simulink model "examples_from_book"  (R2023b)
settings: Solver=ode4  StartTime=0.0  StopTime=0.16  MaxStep=1e-6  RelTol=1e-4  AbsTol=1e-6
libraries: spsParallelRLCBranchLib x20, spsIGBTDiodeLib x6, spsGroundLib x5, spsThreePhaseVIMeasurementLib x3, spsTriangleGeneratorLib x3, spsCurrentMeasurementLib x2, spsDCVoltageSourceLib x2, spsVoltageMeasurementLib x2, spsACVoltageSourceLib x1, spsControlledCurrentSourceLib x1, spsPowerLib x1, spsPower3phInstantaneousLib x1
settings Model: Creator=debatir  LastModifiedBy=debatir
settings SolverCC: SolverResetMethod=Robust

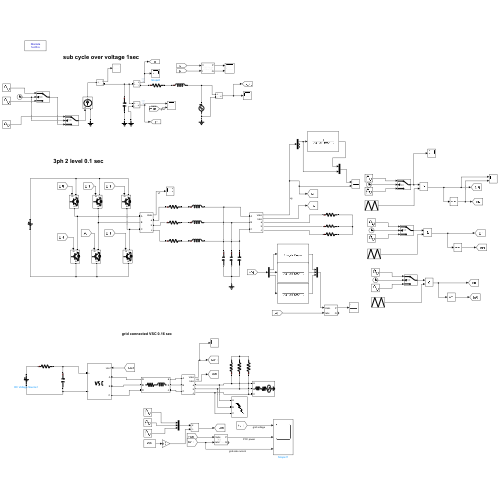
[thumbnail: Simulink's stored preview of the top-level diagram]
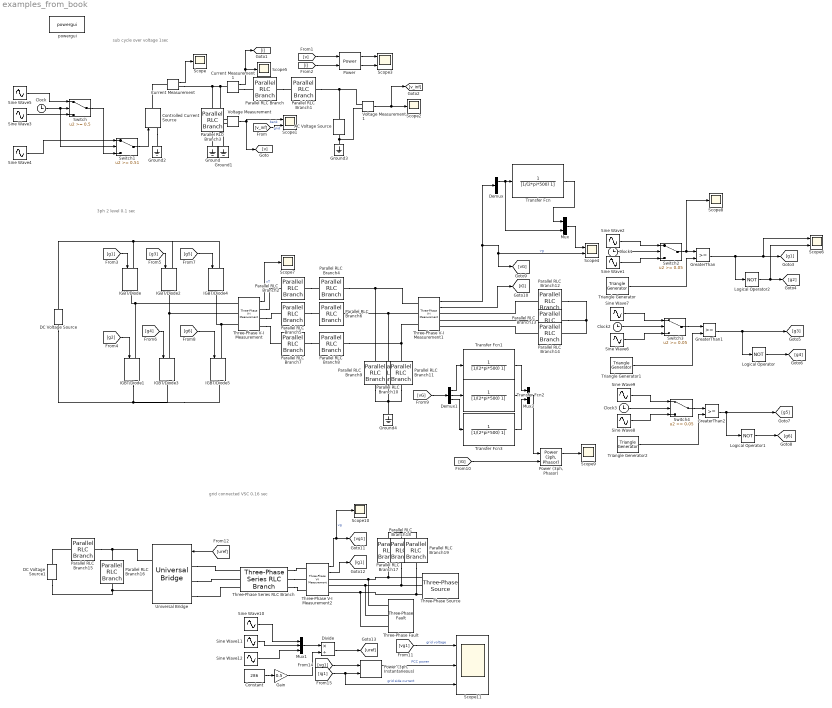
== system examples_from_book ==
  note: grid connected VSC 0.16 sec
  note: 3ph 2 level 0.1 sec
  note: sub cycle over voltage 1sec
  AC Voltage Source : spsACVoltageSourceLib/AC Voltage Source  Amplitude=1  Phase=0  Frequency=60  SampleTime=50e-6  Measurements=None  BusType=PV  Pref=10e3  Qref=0  Qmin=-inf  Qmax=+inf
  Clock{,1..3} (4 alike) : Clock
  Constant : Constant  Value=286
  Controlled Current Source : spsControlledCurrentSourceLib/Controlled Current Source  Initialize=on  Source_Type=AC  Amplitude=0  Phase=0  Frequency=0  Measurements=None
  Current Measurement : spsCurrentMeasurementLib/Current Measurement  PhasorSimulation=off  OutputType=Complex  PSBequivalent=0
  Current Measurement1 : spsCurrentMeasurementLib/Current Measurement  PhasorSimulation=off  OutputType=Complex  PSBequivalent=0
  DC Voltage Source : spsDCVoltageSourceLib/DC Voltage Source  Amplitude=282  Measurements=None
  DC Voltage Source1 : spsDCVoltageSourceLib/DC Voltage Source  Amplitude=286  Measurements=None
  Demux : Demux  Outputs=3
  Demux1 : Demux  Outputs=3
  Divide : Product  Inputs=*/
  Gain : Gain  Gain=0.5
  GreaterThan : RelationalOperator  OutDataTypeStr=boolean  RndMeth=Simplest  InputSameDT=off
  GreaterThan1 : RelationalOperator  OutDataTypeStr=boolean  RndMeth=Simplest  InputSameDT=off
  GreaterThan2 : RelationalOperator  OutDataTypeStr=boolean  RndMeth=Simplest  InputSameDT=off
  Ground{,1..4} (5 alike) : spsGroundLib/Ground  LConnTagsString=a
  IGBT/Diode{,1..5} (6 alike) : spsIGBTDiodeLib/IGBT//Diode  Ron=1e-3  Rs=1e5  Cs=inf  Measurements=off
  Logical Operator : Logic  Operator=NOT  AllPortsSameDT=off  OutDataTypeStr=boolean
  Logical Operator1 : Logic  Operator=NOT  AllPortsSameDT=off  OutDataTypeStr=boolean
  Logical Operator2 : Logic  Operator=NOT  AllPortsSameDT=off  OutDataTypeStr=boolean
  Mux : Mux  Inputs=2
  Mux1 : Mux  Inputs=3
  Mux3 : Mux  Inputs=3
  Parallel RLC Branch : spsParallelRLCBranchLib/Parallel RLC Branch  LConnTagsString=a  RConnTagsString=__new0  BranchType=R  Resistance=0.05  Inductance=0.05  SetiL0=off  InitialCurrent=0  Capacitance=1e-6  Setx0=off  InitialVoltage=0  Measurements=None
  Parallel RLC Branch1 : spsParallelRLCBranchLib/Parallel RLC Branch  LConnTagsString=a  RConnTagsString=__new0  BranchType=L  Resistance=1  Inductance=0.5/(2*pi*60)  SetiL0=off  InitialCurrent=0  Capacitance=1e-6  Setx0=off  InitialVoltage=0  Measurements=None
  Parallel RLC Branch10 : spsParallelRLCBranchLib/Parallel RLC Branch  LConnTagsString=a  RConnTagsString=__new0  BranchType=C  Resistance=1  Inductance=0.2/(2*pi*60)  SetiL0=off  InitialCurrent=0  Capacitance=30e-6  Setx0=off  InitialVoltage=0  Measurements=None
  Parallel RLC Branch11 : spsParallelRLCBranchLib/Parallel RLC Branch  LConnTagsString=a  RConnTagsString=__new0  BranchType=C  Resistance=1  Inductance=0.2/(2*pi*60)  SetiL0=off  InitialCurrent=0  Capacitance=30e-6  Setx0=off  InitialVoltage=0  Measurements=None
  Parallel RLC Branch{12..14,17..19} (6 alike) : spsParallelRLCBranchLib/Parallel RLC Branch  LConnTagsString=a  RConnTagsString=__new0  BranchType=R  Resistance=1  Inductance=0.05  SetiL0=off  InitialCurrent=0  Capacitance=1e-6  Setx0=off  InitialVoltage=0  Measurements=None
  Parallel RLC Branch15 : spsParallelRLCBranchLib/Parallel RLC Branch  LConnTagsString=a  RConnTagsString=__new0  BranchType=R  Resistance=0.05  Inductance=0.05  SetiL0=off  InitialCurrent=0  Capacitance=1e-6  Setx0=off  InitialVoltage=0  Measurements=None
  Parallel RLC Branch16 : spsParallelRLCBranchLib/Parallel RLC Branch  LConnTagsString=a  RConnTagsString=__new0  BranchType=C  Resistance=1  Inductance=0.2/(2*pi*60)  SetiL0=off  InitialCurrent=0  Capacitance=0.09  Setx0=off  InitialVoltage=0  Measurements=None
  Parallel RLC Branch2 : spsParallelRLCBranchLib/Parallel RLC Branch  LConnTagsString=a  RConnTagsString=__new0  BranchType=R  Resistance=0.02  Inductance=0.05  SetiL0=off  InitialCurrent=0  Capacitance=1e-6  Setx0=off  InitialVoltage=0  Measurements=None
  Parallel RLC Branch3 : spsParallelRLCBranchLib/Parallel RLC Branch  LConnTagsString=a  RConnTagsString=__new0  BranchType=C  Resistance=1  Inductance=0.2/(2*pi*60)  SetiL0=off  InitialCurrent=0  Capacitance=0.2/(2*pi*60)  Setx0=off  InitialVoltage=0  Measurements=None
  Parallel RLC Branch4 : spsParallelRLCBranchLib/Parallel RLC Branch  LConnTagsString=a  RConnTagsString=__new0  BranchType=L  Resistance=1  Inductance=0.003  SetiL0=off  InitialCurrent=0  Capacitance=1e-6  Setx0=off  InitialVoltage=0  Measurements=None
  Parallel RLC Branch5 : spsParallelRLCBranchLib/Parallel RLC Branch  LConnTagsString=a  RConnTagsString=__new0  BranchType=R  Resistance=0.02  Inductance=0.05  SetiL0=off  InitialCurrent=0  Capacitance=1e-6  Setx0=off  InitialVoltage=0  Measurements=None
  Parallel RLC Branch6 : spsParallelRLCBranchLib/Parallel RLC Branch  LConnTagsString=a  RConnTagsString=__new0  BranchType=L  Resistance=1  Inductance=0.003  SetiL0=off  InitialCurrent=0  Capacitance=1e-6  Setx0=off  InitialVoltage=0  Measurements=None
  Parallel RLC Branch7 : spsParallelRLCBranchLib/Parallel RLC Branch  LConnTagsString=a  RConnTagsString=__new0  BranchType=R  Resistance=0.02  Inductance=0.05  SetiL0=off  InitialCurrent=0  Capacitance=1e-6  Setx0=off  InitialVoltage=0  Measurements=None
  Parallel RLC Branch8 : spsParallelRLCBranchLib/Parallel RLC Branch  LConnTagsString=a  RConnTagsString=__new0  BranchType=L  Resistance=1  Inductance=0.003  SetiL0=off  InitialCurrent=0  Capacitance=1e-6  Setx0=off  InitialVoltage=0  Measurements=None
  Parallel RLC Branch9 : spsParallelRLCBranchLib/Parallel RLC Branch  LConnTagsString=a  RConnTagsString=__new0  BranchType=C  Resistance=1  Inductance=0.2/(2*pi*60)  SetiL0=off  InitialCurrent=0  Capacitance=30e-6  Setx0=off  InitialVoltage=0  Measurements=None
  Power : spsPowerLib/Power  Freq=60  Vinit=[1, 0]  Iinit=[1, 0]  Ts=0
  "Power (3ph, Instantaneous)" : spsPower3phInstantaneousLib/Power (3ph, Instantaneous)
  "Power (3ph, Phasor)" : spsPower3phPhasorLib/Power (3ph, Phasor)
      settings: LibrarySourceBlock=|
      | sps_lib/Sensors and Measurements/Power
      | (3ph, Phasor)
  Scope{,2,5,7..10} (7 alike) : Scope
  Scope{1,3..4,6} (4 alike) : Scope  NumInputPorts=2
  Scope11 : Scope  NumInputPorts=3
  Sine Wave1 : Sin  Frequency=376.991118  SampleTime=1e-6
  Sine Wave10 : Sin  Amplitude=163  Frequency=376.991118  SampleTime=1e-6
  Sine Wave11 : Sin  Amplitude=163  Frequency=376.991118  Phase=4.18879  SampleTime=1e-6
  Sine Wave12 : Sin  Amplitude=163  Frequency=376.991118  Phase=(2*pi)/3  SampleTime=1e-6
  Sine Wave2 : Sin  Amplitude=.8  Frequency=376.991118  SampleTime=1e-6
  Sine Wave3 : Sin  Frequency=376.991118  SampleTime=50e-6
  Sine Wave4 : Sin  Amplitude=0  Frequency=376.991118  SampleTime=50e-6
  Sine Wave5 : Sin  Amplitude=0.5  Frequency=376.991118  SampleTime=50e-6
  Sine Wave6 : Sin  Frequency=376.991118  Phase=4.18879  SampleTime=1e-6
  Sine Wave7 : Sin  Amplitude=.8  Frequency=376.991118  Phase=4.18879  SampleTime=1e-6
  Sine Wave8 : Sin  Frequency=376.991118  Phase=(2*pi)/3  SampleTime=1e-6
  Sine Wave9 : Sin  Amplitude=.8  Frequency=376.991118  Phase=(2*pi)/3  SampleTime=1e-6
  Switch : Switch  Threshold=0.5  SaturateOnIntegerOverflow=off  InputSameDT=off
  Switch1 : Switch  Threshold=0.51  SaturateOnIntegerOverflow=off  InputSameDT=off
  Switch2 : Switch  Threshold=0.05  SaturateOnIntegerOverflow=off  InputSameDT=off
  Switch3 : Switch  Threshold=0.05  SaturateOnIntegerOverflow=off  InputSameDT=off
  Switch4 : Switch  Threshold=0.05  SaturateOnIntegerOverflow=off  InputSameDT=off
  Three-Phase Series RLC Branch : spsThreePhaseSeriesRLCBranchLib/Three-Phase Series RLC Branch  LConnTagsString=A|B|C  RConnTagsString=A|B|C  BranchType=RL  Resistance=0.016  Inductance=0.2122e-3  Capacitance=1e-6  Measurements=None
  Three-Phase V-I Measurement : spsThreePhaseVIMeasurementLib/Three-Phase V-I Measurement  VoltageMeasurement=phase-to-ground  SetLabelV=off  LabelV=Vabc  Vpu=off  VpuLL=off  CurrentMeasurement=no  SetLabelI=off  LabelI=Iabc  Ipu=off  Pbase=100e6  Vbase=500e3  OutputType=Complex  PhasorSimulation=off  PSBequivalent=0
  Three-Phase V-I Measurement1 : spsThreePhaseVIMeasurementLib/Three-Phase V-I Measurement  VoltageMeasurement=phase-to-ground  SetLabelV=off  LabelV=Vabc  Vpu=off  VpuLL=off  CurrentMeasurement=yes  SetLabelI=off  LabelI=Iabc  Ipu=off  Pbase=100e6  Vbase=500e3  OutputType=Complex  PhasorSimulation=off  PSBequivalent=0
  Three-Phase V-I Measurement2 : spsThreePhaseVIMeasurementLib/Three-Phase V-I Measurement  VoltageMeasurement=phase-to-ground  SetLabelV=off  LabelV=Vabc  Vpu=off  VpuLL=off  CurrentMeasurement=yes  SetLabelI=off  LabelI=Iabc  Ipu=off  Pbase=10e6  Vbase=400  OutputType=Complex  PhasorSimulation=off  PSBequivalent=0
  Three-Phase Fault : spsThreePhaseFaultLib/Three-Phase Fault  InitialStates=0  FaultA=on  FaultB=on  FaultC=on  GroundFault=on  SwitchTimes="[0.05  0.05+3/60]"  External=off  SwitchStatus=NaN  FaultResistance=0.001  GroundResistance=0.01  SnubberResistance=1e6  SnubberCapacitance=inf  Measurements=None
  Three-Phase Source : spsThreePhaseSourceLib/Three-Phase Source  InternalConnection=Yg  VoltagePhases=off  Voltage=175  PhaseAngle=0  Voltage_phases=[25e3 25e3 25e3]/sqrt(3)  PhaseAngles_phases=[0 -120 +120]  Frequency=60  NonIdealSource=on  SpecifyImpedance=off  Resistance=1.6  Inductance=16.58e-3  ShortCircuitLevel=100e6  BaseVoltage=25e3  XRratio=7  BusType=swing  Pref=10e3  Qref=0  Prefabc=[10e3, 10e3, 10e3]  Qrefabc=[0, 0, 0]  Qmin=-inf  Qmax=inf
  Transfer Fcn{,1..3} (4 alike) : TransferFcn  Numerator=[0 1]  Denominator=[1/(2*pi*500) 1]
  Triangle Generator : spsTriangleGeneratorLib/Triangle Generator  Freq=1980  Phase=0  Ts=1e-6
  Triangle Generator1 : spsTriangleGeneratorLib/Triangle Generator  Freq=1980  Phase=0  Ts=1e-6
  Triangle Generator2 : spsTriangleGeneratorLib/Triangle Generator  Freq=1980  Phase=0  Ts=1e-6
  Universal Bridge : spsUniversalBridgeLib/Universal Bridge  Arms=3  SnubberResistance=1e5  SnubberCapacitance=inf  Device=Average-model based VSC  Ron=1e-3  Lon=0  ForwardVoltages="[  0  0  ]"  ForwardVoltage=0  GTOparameters=[ 10e-6 , 20e-6 ]  IGBTparameters=[ 1e-6 , 2e-6 ]  Measurements=None  Measurements_2=None  converterType=Rectifier
  Voltage Measurement : spsVoltageMeasurementLib/Voltage Measurement  PhasorSimulation=off  OutputType=Complex  PSBequivalent=0
  Voltage Measurement1 : spsVoltageMeasurementLib/Voltage Measurement  PhasorSimulation=off  OutputType=Complex  PSBequivalent=0
  powergui : sps_lib/powergui  Priority=1  SimulationMode=Discrete  SampleTime=1e-6  frequency=60  Iterations=50  frequencyindice=0  Pbase=100e6  ErrMax=1e-4  UnitsV=kV  UnitsW=MW  buscounter=0  FunctionMessages=off  echomessages=off  EnableUseOfTLC=off  CurrentSourceSwitches=off  DisableSnubberDevices=off  DisableRonSwitches=off  DisableVfSwitches=off  DisplayEquations=off  AutomaticDiscreteSolvers=off  SolverType=Tustin  Interpol=off  ExternalGateDelay=off  methode=off  Ts=100  x0status=blocks  SPID=on  SwTol=0  HookPort=off  NonlinearTolerance=1e-4  nMaxIteration=100  ContinueOnMaxIteration=off  RestoreLinks=warning  ResistiveCurrentMeasurement=off  Frange=[0:2:500]  Ylog=off  Xlog=on  ShowGrid=off  save=off  variable=ZData  structure=0  ZoomFFT=off  StartTime=0.0  cycles=1  DisplayStyle=1  fundamental=60  FreqAxis=off  MaxFrequency=1000  frequencyindicesteady=1  RmsSteady=1  display=off
  wires:
  Current Measurement/1 -> Scope/1
  Voltage Measurement/1 -> [v], Scope1/1  "bank"
  [v_inf] -> Scope1/2  "grid"
  Voltage Measurement1/1 -> [v_inf], Scope2/1
  [v] -> Power/1
  [i] -> Power/2
  Power/1 -> Scope3/1
  Power/2 -> Scope3/2
  Current Measurement1/1 -> [i], Scope5/1
  Clock/1 -> Switch1/2, Switch/2
  Sine Wave5/1 -> Switch/1
  Sine Wave3/1 -> Switch/3
  Switch1/1 -> Controlled Current Source/1
  Switch/1 -> Switch1/3
  Sine Wave4/1 -> Switch1/1
  Sine Wave1/1 -> Switch2/3
  Clock1/1 -> Switch2/2
  Sine Wave2/1 -> Switch2/1
  Triangle Generator/1 -> GreaterThan/2
  GreaterThan/1 -> Logical Operator2/1, Scope6/1, [g1]
  Logical Operator2/1 -> Scope6/2, [g2]
  Logical Operator/1 -> [g4]
  GreaterThan1/1 -> Logical Operator/1, [g3]
  Triangle Generator1/1 -> GreaterThan1/2
  Sine Wave7/1 -> Switch3/1
  Clock2/1 -> Switch3/2
  Sine Wave6/1 -> Switch3/3
  Sine Wave8/1 -> Switch4/3
  Clock3/1 -> Switch4/2
  Sine Wave9/1 -> Switch4/1
  Switch4/1 -> GreaterThan2/1
  Triangle Generator2/1 -> GreaterThan2/2
  GreaterThan2/1 -> [g5], Logical Operator1/1
  Logical Operator1/1 -> [g6]
  [g1] -> IGBT/Diode/1
  [g2] -> IGBT/Diode1/1
  [g3] -> IGBT/Diode2/1
  [g4] -> IGBT/Diode3/1
  [g5] -> IGBT/Diode4/1
  [g6] -> IGBT/Diode5/1
  Three-Phase V-I Measurement1/1 -> Demux/1, [vG], Scope4/2  "vg"
  Three-Phase V-I Measurement/1 -> Scope7/1  "vT"
  Switch3/1 -> GreaterThan1/1
  Switch2/1 -> Scope8/1, GreaterThan/1
  Three-Phase V-I Measurement1/2 -> [iG]
  [iG] -> "Power (3ph, Phasor)"/2
  "Power (3ph, Phasor)"/1 -> Scope9/1
  Demux/1 -> Mux/2, Transfer Fcn/1
  Transfer Fcn/1 -> Mux/1
  Mux/1 -> Scope4/1
  Three-Phase V-I Measurement2/2 -> [ig1]
  Three-Phase V-I Measurement2/1 -> Scope10/1, [vg1]  "vg"
  Constant/1 -> Gain/1
  Gain/1 -> Divide/2
  Divide/1 -> [uref]
  [uref] -> Universal Bridge/1
  Mux1/1 -> Divide/1
  Sine Wave10/1 -> Mux1/1
  Sine Wave11/1 -> Mux1/2
  Sine Wave12/1 -> Mux1/3
  [vg1] -> Scope11/1  "grid voltage"
  [vg1] -> "Power (3ph, Instantaneous)"/1
  [ig1] -> Scope11/3, "Power (3ph, Instantaneous)"/2  "grid side current"
  [vG] -> Demux1/1
  Demux1/1 -> Transfer Fcn1/1
  Demux1/2 -> Transfer Fcn2/1
  Demux1/3 -> Transfer Fcn3/1
  Transfer Fcn2/1 -> Mux3/2
  Transfer Fcn1/1 -> Mux3/1
  Transfer Fcn3/1 -> Mux3/3
  Mux3/1 -> "Power (3ph, Phasor)"/1
  "Power (3ph, Instantaneous)"/1 -> Scope11/2  "PCC power"
  connections:
  Parallel RLC Branch/RConn1 -- Parallel RLC Branch1/LConn1
  Current Measurement/RConn1 -- Parallel RLC Branch3/LConn1 -- Current Measurement1/LConn1 -- Voltage Measurement/LConn1
  Controlled Current Source/RConn1 -- Current Measurement/LConn1
  Ground/LConn1 -- Parallel RLC Branch3/RConn1
  Ground1/LConn1 -- Voltage Measurement/LConn2
  Controlled Current Source/LConn1 -- Ground2/LConn1
  Parallel RLC Branch1/RConn1 -- Voltage Measurement1/LConn1 -- AC Voltage Source/RConn1
  Ground3/LConn1 -- Voltage Measurement1/LConn2 -- AC Voltage Source/LConn1
  Current Measurement1/RConn1 -- Parallel RLC Branch/LConn1
  Three-Phase V-I Measurement/LConn1 -- IGBT/Diode1/LConn1 -- IGBT/Diode/RConn1
  Three-Phase V-I Measurement/LConn2 -- IGBT/Diode3/LConn1 -- IGBT/Diode2/RConn1
  Three-Phase V-I Measurement/LConn3 -- IGBT/Diode5/LConn1 -- IGBT/Diode4/RConn1
  DC Voltage Source/RConn1 -- IGBT/Diode4/LConn1 -- IGBT/Diode2/LConn1 -- IGBT/Diode/LConn1
  DC Voltage Source/LConn1 -- IGBT/Diode5/RConn1 -- IGBT/Diode3/RConn1 -- IGBT/Diode1/RConn1
  Parallel RLC Branch2/RConn1 -- Parallel RLC Branch4/LConn1
  Parallel RLC Branch5/RConn1 -- Parallel RLC Branch6/LConn1
  Parallel RLC Branch7/RConn1 -- Parallel RLC Branch8/LConn1
  Three-Phase V-I Measurement/RConn2 -- Parallel RLC Branch5/LConn1
  Three-Phase V-I Measurement/RConn1 -- Parallel RLC Branch2/LConn1
  Three-Phase V-I Measurement/RConn3 -- Parallel RLC Branch7/LConn1
  Parallel RLC Branch9/RConn1 -- Parallel RLC Branch11/RConn1 -- Ground4/LConn1 -- Parallel RLC Branch10/RConn1
  Three-Phase V-I Measurement1/LConn2 -- Parallel RLC Branch6/RConn1 -- Parallel RLC Branch10/LConn1
  Parallel RLC Branch4/RConn1 -- Parallel RLC Branch9/LConn1 -- Three-Phase V-I Measurement1/LConn1
  Parallel RLC Branch8/RConn1 -- Parallel RLC Branch11/LConn1 -- Three-Phase V-I Measurement1/LConn3
  Parallel RLC Branch12/LConn1 -- Three-Phase V-I Measurement1/RConn1
  Parallel RLC Branch13/LConn1 -- Three-Phase V-I Measurement1/RConn2
  Parallel RLC Branch14/LConn1 -- Three-Phase V-I Measurement1/RConn3
  Parallel RLC Branch12/RConn1 -- Parallel RLC Branch13/RConn1 -- Parallel RLC Branch14/RConn1
  Parallel RLC Branch15/RConn1 -- Parallel RLC Branch16/LConn1 -- Universal Bridge/RConn1
  DC Voltage Source1/LConn1 -- Parallel RLC Branch16/RConn1 -- Universal Bridge/RConn2
  DC Voltage Source1/RConn1 -- Parallel RLC Branch15/LConn1
  Universal Bridge/LConn1 -- Three-Phase Series RLC Branch/LConn1
  Universal Bridge/LConn2 -- Three-Phase Series RLC Branch/LConn2
  Universal Bridge/LConn3 -- Three-Phase Series RLC Branch/LConn3
  Three-Phase Series RLC Branch/RConn2 -- Three-Phase V-I Measurement2/LConn2
  Three-Phase Series RLC Branch/RConn1 -- Three-Phase V-I Measurement2/LConn1
  Three-Phase Series RLC Branch/RConn3 -- Three-Phase V-I Measurement2/LConn3
  Three-Phase Source/RConn1 -- Parallel RLC Branch17/LConn1 -- Three-Phase Fault/LConn1 -- Three-Phase V-I Measurement2/RConn1
  Three-Phase Source/RConn2 -- Parallel RLC Branch18/LConn1 -- Three-Phase Fault/LConn2 -- Three-Phase V-I Measurement2/RConn2
  Three-Phase Source/RConn3 -- Parallel RLC Branch19/LConn1 -- Three-Phase Fault/LConn3 -- Three-Phase V-I Measurement2/RConn3
  Parallel RLC Branch17/RConn1 -- Parallel RLC Branch18/RConn1 -- Parallel RLC Branch19/RConn1
